simulink model "Simulink_electronico"  (R2024a)
settings: Solver=VariableStepAuto  StartTime=0.0  StopTime=.001  RelTol=1e-3
values from neighbouring files (symbols this model uses):
  C = 0.0000001    (= 1e-07)    [Ec4.m]    (also in Smulink_datos.m)
  L = 0.004    [Ec4.m]    (also in Smulink_datos.m)
  R = 120    [Ec4.m]    (also in Smulink_datos.m)
settings Model: Creator=Braulio Ramíreza  LastModifiedBy=Braulio Ramíreza

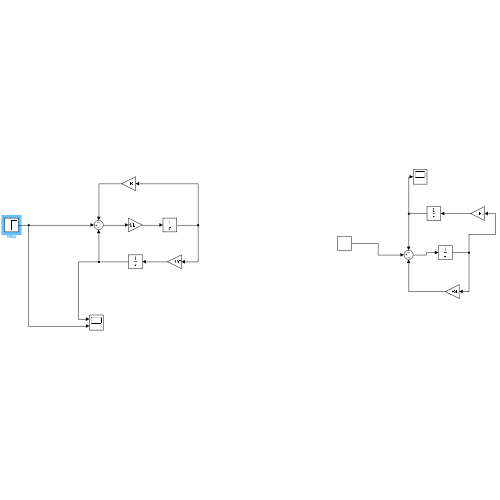
[thumbnail: Simulink's stored preview of the top-level diagram]
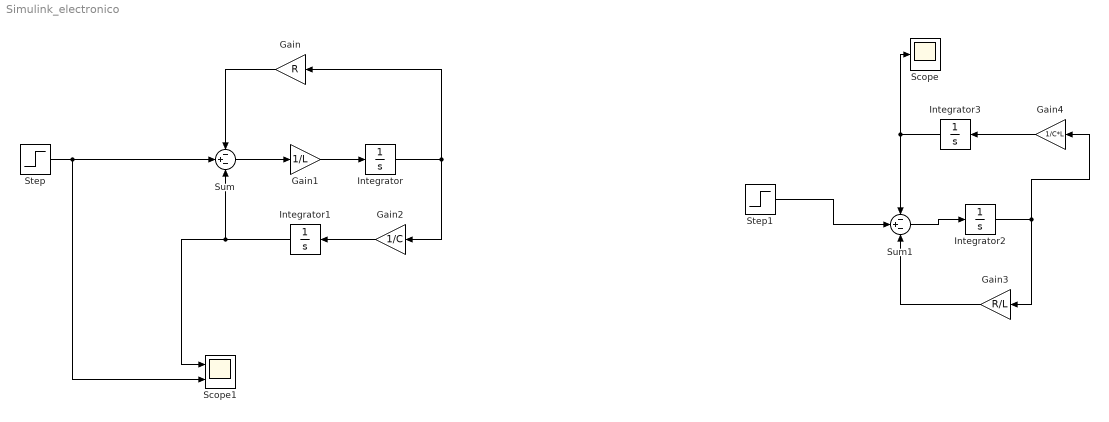
== system Simulink_electronico ==
  Gain : Gain  Gain=R
  Gain1 : Gain  Gain=1/L
  Gain2 : Gain  Gain=1/C
  Gain3 : Gain  Gain=R/L
  Gain4 : Gain  Gain=1/C*L
  Integrator{,1..3} (4 alike) : Integrator
  Scope : Scope
  Scope1 : Scope  NumInputPorts=2
  Step : Step  Time=0  After=5  SampleTime=0
  Step1 : Step  Time=0  After=5  SampleTime=0
  Sum : Sum  Inputs=-+-
  Sum1 : Sum  Inputs=-+-
  wires:
  Step/1 -> Scope1/2, Sum/2
  Gain/1 -> Sum/1
  Sum/1 -> Gain1/1
  Gain1/1 -> Integrator/1
  Gain2/1 -> Integrator1/1
  Integrator1/1 -> Scope1/1, Sum/3
  Integrator/1 -> Gain2/1, Gain/1
  Sum1/1 -> Integrator2/1
  Integrator2/1 -> Gain3/1, Gain4/1
  Gain3/1 -> Sum1/3
  Gain4/1 -> Integrator3/1
  Step1/1 -> Sum1/2
  Integrator3/1 -> Sum1/1, Scope/1
